simulink subsystem "SWs"  (R2023a)
settings: Solver=VariableStepAuto  StartTime=0.0  StopTime=10.0  RelTol=1e-3
undefined symbols (not defined in the file or in its folder): samplingTime
libraries: stm32f4xxblockslib x2
settings Model: Creator=JesseJabezArendse  LastModifiedBy=JesseJabezArendse

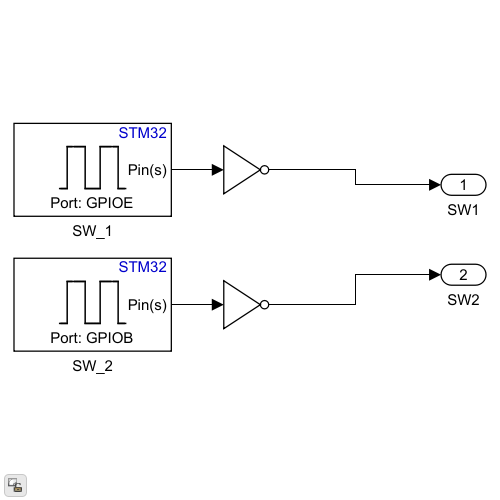
[thumbnail: Simulink's stored preview of the top-level diagram]
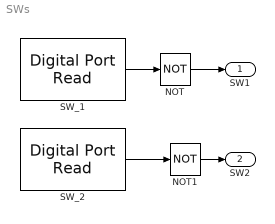
== system SWs ==
  NOT : Logic  Operator=NOT  IconShape=distinctive  AllPortsSameDT=off  OutDataTypeStr=boolean
  NOT1 : Logic  Operator=NOT  IconShape=distinctive  AllPortsSameDT=off  OutDataTypeStr=boolean
  SW_1 : stm32f4xxblockslib/Digital Port Read  PortName=GPIOE  PinNumber=[6]  ReadOperation=on  IOAsArray=on  SampleTime=samplingTime  EnableSimPort=off
      settings: LibrarySourceBlock=stm32l4xxblockslib/Digital Port Read
  SW_2 : stm32f4xxblockslib/Digital Port Read  PortName=GPIOB  PinNumber=[2]  ReadOperation=on  IOAsArray=on  SampleTime=samplingTime  EnableSimPort=off
      settings: LibrarySourceBlock=stm32l4xxblockslib/Digital Port Read
  SW1 : Outport
  SW2 : Outport  Port=2
  wires:
  SW_1/1 -> NOT/1
  SW_2/1 -> NOT1/1
  NOT/1 -> SW1/1
  NOT1/1 -> SW2/1
